simulink model "Mooventure2016_Rev5"  (Simulink 7.7)
settings: Solver=FixedStepDiscrete  StartTime=0.0  StopTime=10  RelTol=1e-3
PreLoadFcn:
  | try, eval([bdroot '_setup']); catch, eval('model_setup', ''); end
InitFcn:
  | try, eval([bdroot '_setup']); catch, eval('model_setup', ''); end
undefined symbols (not defined in the file): ECM, H1, motohawk_build_version, motohawk_trunc_name, motohawk_vardec_config_group, motohawk_vardec_path, xD
libraries: MotoHawk_lib x976, motohawk_control_primitives_lib x41, simulink x27, motohawk_annotations_lib x3
(part 2 of 16)

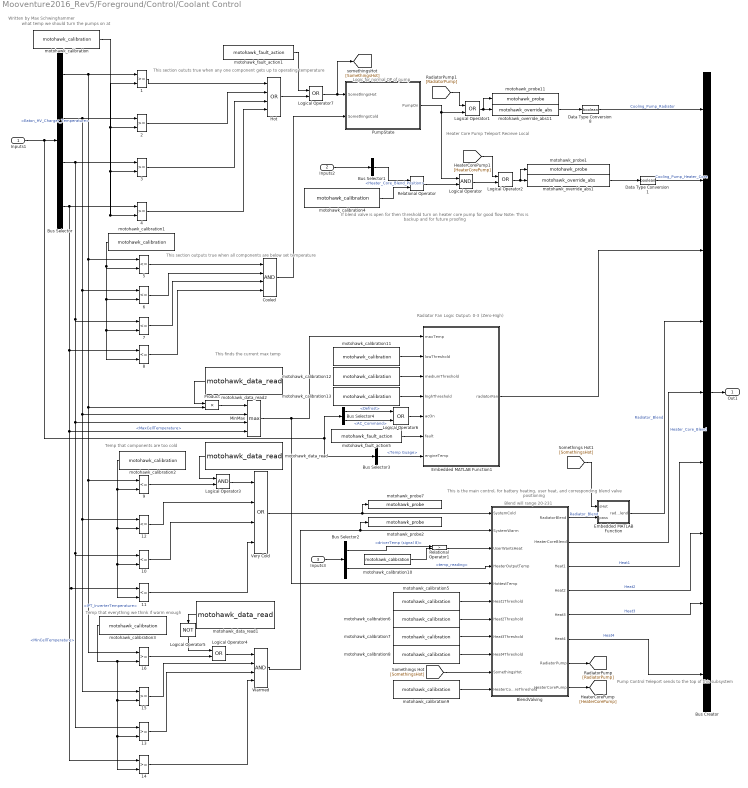
== system Mooventure2016_Rev5/Foreground/Control/Coolant Control ==
  note: This finds the current max temp
  note: Blend will range 20-231
  note: This is the main control, for battery heating, user heat,
      |  and corresponding blend valve positioning
  note: Temp that everything we think if warm enough
  note: Temp that components are too cold
  note: This section outputs true when all components
      | are below set temperature
  note: what temp we should turn the pumps on at
  note: This section oututs true when any one component
      | gets up to operating temperature
  note: Logic for normal OP of pump
  note: If blend valve is open for then threshold turn on heater
      | core pump for good flow
      | Note: This is backup and for future proofing
  note: Heater Core Pump Teleport Recieve Local
  note: Radiator Fan Logic
      | Output: 0-3 (Zero-High)
  note: Pump Control Teleport sends to the top of this subsystem
  note: Written by Max Schwinghammer
  Inputs1 : Inport
  Inputs2 : Inport  Port=2
  Inputs3 : Inport  Port=3
  {1..4,13..16} (8 alike) : RelationalOperator  OutDataTypeStr=boolean
  {5..12} (8 alike) : RelationalOperator  Operator=<=  OutDataTypeStr=boolean
  BlendValving : Stateflow chart  TreatAsAtomicUnit=on
  Bus Creator : BusCreator  Inputs=9
  Bus Selector : BusSelector  OutputSignals=Eaton_Charger.Eaton_Charger.Eaton_HV_Charger_Temperature,IPT.ID 278 IPT Status 1.IPT_InverterTemperature,Battery_Inputs.MinCellTemperature,Battery_Inputs.MaxCellTemperature
  Bus Selector1 : BusSelector  OutputSignals=Analog_Inputs.Coolant.Heater_Core_Blend_Position
  Bus Selector2 : BusSelector  OutputSignals=Driver Inputs.driverTemp (signal 8),Analog_Inputs.Coolant.temp_reading
  Bus Selector3 : BusSelector  OutputSignals=Engine Inputs.Temp Guage
  Bus Selector4 : BusSelector  OutputSignals=CAN Gateway.Defrost,CAN Gateway.AC_Command
  Cooled : Logic  Inputs=4  AllPortsSameDT=off  OutDataTypeStr=boolean
  Data Type Conversion1 : DataTypeConversion  OutDataTypeStr=boolean
  Data Type Conversion8 : DataTypeConversion  OutDataTypeStr=boolean
  Embedded MATLAB Function : Stateflow chart  TreatAsAtomicUnit=on
  Embedded MATLAB Function1 : Stateflow chart  TreatAsAtomicUnit=on
  Hot : Logic  Operator=OR  Inputs=4  AllPortsSameDT=off  OutDataTypeStr=boolean
  Logical Operator : Logic  AllPortsSameDT=off  OutDataTypeStr=boolean
  Logical Operator{1..2,4,6..7} (5 alike) : Logic  Operator=OR  AllPortsSameDT=off  OutDataTypeStr=boolean
  Logical Operator3 : Logic  AllPortsSameDT=off  OutDataTypeStr=boolean
  Logical Operator5 : Logic  Operator=NOT  Inputs=1  AllPortsSameDT=off  OutDataTypeStr=boolean
  MinMax : MinMax  Function=max  Inputs=4
  Product : Product  RndMeth=Zero
  PumpState : Stateflow chart  TreatAsAtomicUnit=on
  Relational Operator : RelationalOperator  OutDataTypeStr=boolean
  Relational Operator1 : RelationalOperator  Operator=>  OutDataTypeStr=boolean
  Very Cold : Logic  Operator=OR  Inputs=4  AllPortsSameDT=off  OutDataTypeStr=boolean
  Warmed : Logic  Inputs=4  AllPortsSameDT=off  OutDataTypeStr=boolean
  motohawk_calibration : MotoHawk_lib/Calibration & Probing Blocks/motohawk_calibration  nam='Pump_On_Temp'  val=30  storage=Calibration  show_more=off  name_source=Use Parameter  data_type=Inherit from 'Default Value'  read_level=1  write_level=1  ovr_cals=on  view_as=Number  enum_struct={'Disabled', 'Enabled'}  vector_style=Wide Row  use_help_units=off  help=''  units=''  use_header_enum=off  row_header_enum={}  col_header_enum={}  use_min_max=off  min_val=-inf  max_val=inf  use_precision=off  precision=''  gain=1  offset=0  exp=1  use_mototune_group=off  mototune_group=motohawk_vardec_path(gcb)
  motohawk_calibration1 : MotoHawk_lib/Calibration & Probing Blocks/motohawk_calibration  nam='Pump_Off_Temp'  val=25  storage=Calibration  show_more=off  name_source=Use Parameter  data_type=Inherit from 'Default Value'  read_level=1  write_level=1  ovr_cals=on  view_as=Number  enum_struct={'Disabled', 'Enabled'}  vector_style=Wide Row  use_help_units=off  help=''  units=''  use_header_enum=off  row_header_enum={}  col_header_enum={}  use_min_max=off  min_val=-inf  max_val=inf  use_precision=off  precision=''  gain=1  offset=0  exp=1  use_mototune_group=off  mototune_group=motohawk_vardec_path(gcb)
  motohawk_calibration10 : MotoHawk_lib/Calibration & Probing Blocks/motohawk_calibration  nam='Heat_On_Driver_Threshold'  val=72  storage=Calibration  show_more=off  name_source=Use Parameter  data_type=Inherit from 'Default Value'  read_level=1  write_level=1  ovr_cals=on  view_as=Number  enum_struct={'Disabled', 'Enabled'}  vector_style=Wide Row  use_help_units=off  help=''  units=''  use_header_enum=off  row_header_enum={}  col_header_enum={}  use_min_max=off  min_val=-inf  max_val=inf  use_precision=off  precision=''  gain=1  offset=0  exp=1  use_mototune_group=off  mototune_group=motohawk_vardec_path(gcb)
  motohawk_calibration11 : MotoHawk_lib/Calibration & Probing Blocks/motohawk_calibration  nam='Low_Threshold'  val=40  storage=Calibration  show_more=on  name_source=Use Parameter  data_type=double  read_level=1  write_level=1  ovr_cals=on  view_as=Number  enum_struct={'Disabled', 'Enabled'}  vector_style=Wide Row  use_help_units=off  help=''  units=''  use_header_enum=off  row_header_enum={}  col_header_enum={}  use_min_max=off  min_val=-inf  max_val=inf  use_precision=off  precision=''  gain=1  offset=0  exp=1  use_mototune_group=off  mototune_group=motohawk_vardec_path(gcb)
  motohawk_calibration12 : MotoHawk_lib/Calibration & Probing Blocks/motohawk_calibration  nam='Medium_Threshold'  val=50  storage=Calibration  show_more=on  name_source=Use Parameter  data_type=double  read_level=1  write_level=1  ovr_cals=on  view_as=Number  enum_struct={'Disabled', 'Enabled'}  vector_style=Wide Row  use_help_units=off  help=''  units=''  use_header_enum=off  row_header_enum={}  col_header_enum={}  use_min_max=off  min_val=-inf  max_val=inf  use_precision=off  precision=''  gain=1  offset=0  exp=1  use_mototune_group=off  mototune_group=motohawk_vardec_path(gcb)
  motohawk_calibration13 : MotoHawk_lib/Calibration & Probing Blocks/motohawk_calibration  nam='High_Threshold'  val=65  storage=Calibration  show_more=on  name_source=Use Parameter  data_type=double  read_level=1  write_level=1  ovr_cals=on  view_as=Number  enum_struct={'Disabled', 'Enabled'}  vector_style=Wide Row  use_help_units=off  help=''  units=''  use_header_enum=off  row_header_enum={}  col_header_enum={}  use_min_max=off  min_val=-inf  max_val=inf  use_precision=off  precision=''  gain=1  offset=0  exp=1  use_mototune_group=off  mototune_group=motohawk_vardec_path(gcb)
  motohawk_calibration2 : MotoHawk_lib/Calibration & Probing Blocks/motohawk_calibration  nam='Too_Cold_Temp'  val=0  storage=Calibration  show_more=off  name_source=Use Parameter  data_type=Inherit from 'Default Value'  read_level=1  write_level=1  ovr_cals=on  view_as=Number  enum_struct={'Disabled', 'Enabled'}  vector_style=Wide Row  use_help_units=off  help=''  units=''  use_header_enum=off  row_header_enum={}  col_header_enum={}  use_min_max=off  min_val=-inf  max_val=inf  use_precision=off  precision=''  gain=1  offset=0  exp=1  use_mototune_group=off  mototune_group=motohawk_vardec_path(gcb)
  motohawk_calibration3 : MotoHawk_lib/Calibration & Probing Blocks/motohawk_calibration  nam='Warmed_Up_Temp'  val=15  storage=Calibration  show_more=off  name_source=Use Parameter  data_type=Inherit from 'Default Value'  read_level=1  write_level=1  ovr_cals=on  view_as=Number  enum_struct={'Disabled', 'Enabled'}  vector_style=Wide Row  use_help_units=off  help=''  units=''  use_header_enum=off  row_header_enum={}  col_header_enum={}  use_min_max=off  min_val=-inf  max_val=inf  use_precision=off  precision=''  gain=1  offset=0  exp=1  use_mototune_group=off  mototune_group=motohawk_vardec_path(gcb)
  motohawk_calibration4 : MotoHawk_lib/Calibration & Probing Blocks/motohawk_calibration  nam='Blend_Pump_On_Threshold'  val=25  storage=Calibration  show_more=off  name_source=Use Parameter  data_type=Inherit from 'Default Value'  read_level=1  write_level=1  ovr_cals=on  view_as=Number  enum_struct={'Disabled', 'Enabled'}  vector_style=Wide Row  use_help_units=off  help=''  units=''  use_header_enum=off  row_header_enum={}  col_header_enum={}  use_min_max=off  min_val=-inf  max_val=inf  use_precision=off  precision=''  gain=1  offset=0  exp=1  use_mototune_group=off  mototune_group=motohawk_vardec_path(gcb)
  motohawk_calibration5 : MotoHawk_lib/Calibration & Probing Blocks/motohawk_calibration  nam='Heat1_Threshold'  val=-1  storage=Calibration  show_more=off  name_source=Use Parameter  data_type=Inherit from 'Default Value'  read_level=1  write_level=1  ovr_cals=on  view_as=Number  enum_struct={'Disabled', 'Enabled'}  vector_style=Wide Row  use_help_units=off  help=''  units=''  use_header_enum=off  row_header_enum={}  col_header_enum={}  use_min_max=off  min_val=-inf  max_val=inf  use_precision=off  precision=''  gain=1  offset=0  exp=1  use_mototune_group=off  mototune_group=motohawk_vardec_path(gcb)
  motohawk_calibration6 : MotoHawk_lib/Calibration & Probing Blocks/motohawk_calibration  nam='Heat2_Threshold'  val=-5  storage=Calibration  show_more=off  name_source=Use Parameter  data_type=Inherit from 'Default Value'  read_level=1  write_level=1  ovr_cals=on  view_as=Number  enum_struct={'Disabled', 'Enabled'}  vector_style=Wide Row  use_help_units=off  help=''  units=''  use_header_enum=off  row_header_enum={}  col_header_enum={}  use_min_max=off  min_val=-inf  max_val=inf  use_precision=off  precision=''  gain=1  offset=0  exp=1  use_mototune_group=off  mototune_group=motohawk_vardec_path(gcb)
  motohawk_calibration7 : MotoHawk_lib/Calibration & Probing Blocks/motohawk_calibration  nam='Heat3_Threshold'  val=-10  storage=Calibration  show_more=off  name_source=Use Parameter  data_type=Inherit from 'Default Value'  read_level=1  write_level=1  ovr_cals=on  view_as=Number  enum_struct={'Disabled', 'Enabled'}  vector_style=Wide Row  use_help_units=off  help=''  units=''  use_header_enum=off  row_header_enum={}  col_header_enum={}  use_min_max=off  min_val=-inf  max_val=inf  use_precision=off  precision=''  gain=1  offset=0  exp=1  use_mototune_group=off  mototune_group=motohawk_vardec_path(gcb)
  motohawk_calibration8 : MotoHawk_lib/Calibration & Probing Blocks/motohawk_calibration  nam='Heat4_Threshold'  val=-15  storage=Calibration  show_more=off  name_source=Use Parameter  data_type=Inherit from 'Default Value'  read_level=1  write_level=1  ovr_cals=on  view_as=Number  enum_struct={'Disabled', 'Enabled'}  vector_style=Wide Row  use_help_units=off  help=''  units=''  use_header_enum=off  row_header_enum={}  col_header_enum={}  use_min_max=off  min_val=-inf  max_val=inf  use_precision=off  precision=''  gain=1  offset=0  exp=1  use_mototune_group=off  mototune_group=motohawk_vardec_path(gcb)
  motohawk_calibration9 : MotoHawk_lib/Calibration & Probing Blocks/motohawk_calibration  nam='Heater_Core_Threshold'  val=46  storage=Calibration  show_more=off  name_source=Use Parameter  data_type=Inherit from 'Default Value'  read_level=1  write_level=1  ovr_cals=on  view_as=Number  enum_struct={'Disabled', 'Enabled'}  vector_style=Wide Row  use_help_units=off  help=''  units=''  use_header_enum=off  row_header_enum={}  col_header_enum={}  use_min_max=off  min_val=-inf  max_val=inf  use_precision=off  precision=''  gain=1  offset=0  exp=1  use_mototune_group=off  mototune_group=motohawk_vardec_path(gcb)
  motohawk_data_read : MotoHawk_lib/Data Storage Blocks/motohawk_data_read  source=Lookup By Name  structure=Scalar  operation=Read scalar from location by index  sz_vec=4  sz_row=2  sz_col=3  typ=boolean  nam='Eaton_Plugged_In'  checkNull=on  struct_inst_name='MyData'  struct_nam='MyStruct'
  motohawk_data_read1 : MotoHawk_lib/Data Storage Blocks/motohawk_data_read  source=Lookup By Name  structure=Scalar  operation=Read scalar from location by index  sz_vec=4  sz_row=2  sz_col=3  typ=boolean  nam='Eaton_Plugged_In'  checkNull=on  struct_inst_name='MyData'  struct_nam='MyStruct'
  motohawk_data_read2 : MotoHawk_lib/Data Storage Blocks/motohawk_data_read  source=Lookup By Name  structure=Scalar  operation=Read scalar from location by index  sz_vec=4  sz_row=2  sz_col=3  typ=boolean  nam='Eaton_Plugged_In'  checkNull=on  struct_inst_name='MyData'  struct_nam='MyStruct'
  motohawk_fault_action1 : MotoHawk_lib/Fault Management Blocks/motohawk_fault_action  nam='Pump_On'  output_status=on  eval_nam=Pump_On
  motohawk_fault_action5 : MotoHawk_lib/Fault Management Blocks/motohawk_fault_action  nam='Cooling_Max'  output_status=on  eval_nam=Cooling_Max
  motohawk_override_abs1 : MotoHawk_lib/Calibration & Probing Blocks/motohawk_override_abs  SystemSampleTime=-1  parent_name='Cooling_Pump_Heater_Core_Ovr'  parent_val=0  show_more=on  name_source=Use Parameter  parent_read_level=1  parent_override_level=1  view_as=Number  enum_struct={'Disabled', 'Enabled'}  use_help_units=off  parent_help=''  parent_units=''  use_min_max=off  parent_min=-inf  parent_max=inf  use_precision=off  parent_precision=''  parent_gain=1  parent_offset=0  parent_exp=1  use_mototune_group=off  parent_group=motohawk_vardec_path(gcb)
  motohawk_override_abs11 : MotoHawk_lib/Calibration & Probing Blocks/motohawk_override_abs  SystemSampleTime=-1  parent_name='Cooling_Pump_Radiator_Ovr'  parent_val=0  show_more=on  name_source=Use Parameter  parent_read_level=1  parent_override_level=1  view_as=Number  enum_struct={'Disabled', 'Enabled'}  use_help_units=off  parent_help=''  parent_units=''  use_min_max=off  parent_min=-inf  parent_max=inf  use_precision=off  parent_precision=''  parent_gain=1  parent_offset=0  parent_exp=1  use_mototune_group=off  parent_group=motohawk_vardec_path(gcb)
  motohawk_probe1 : MotoHawk_lib/Calibration & Probing Blocks/motohawk_probe  nam='Cooling_Pump_Heater_Core_Probe'  show_more=on  name_source=Use Parameter  read_level=1  view_as=Number  enum_struct={'Disabled', 'Enabled'}  vector_style=Wide Row  use_help_units=off  help=''  units=''  use_header_enum=off  row_header_enum={}  col_header_enum={}  use_precision=off  precision=''  gain=1  offset=0  exp=1  use_mototune_group=off  mototune_group=motohawk_vardec_path(gcb)
  motohawk_probe11 : MotoHawk_lib/Calibration & Probing Blocks/motohawk_probe  nam='Cooling_Pump_Radiator_Probe'  show_more=on  name_source=Use Parameter  read_level=1  view_as=Number  enum_struct={'Disabled', 'Enabled'}  vector_style=Wide Row  use_help_units=off  help=''  units=''  use_header_enum=off  row_header_enum={}  col_header_enum={}  use_precision=off  precision=''  gain=1  offset=0  exp=1  use_mototune_group=off  mototune_group=motohawk_vardec_path(gcb)
  motohawk_probe2 : MotoHawk_lib/Calibration & Probing Blocks/motohawk_probe  nam='System_Warm_Prb'  show_more=off  name_source=Use Parameter  read_level=1  view_as=Number  enum_struct={'Disabled', 'Enabled'}  vector_style=Wide Row  use_help_units=off  help=''  units=''  use_header_enum=off  row_header_enum={}  col_header_enum={}  use_precision=off  precision=''  gain=1  offset=0  exp=1  use_mototune_group=off  mototune_group=motohawk_vardec_path(gcb)
  motohawk_probe7 : MotoHawk_lib/Calibration & Probing Blocks/motohawk_probe  nam='System_Cold_Prb'  show_more=off  name_source=Use Parameter  read_level=1  view_as=Number  enum_struct={'Disabled', 'Enabled'}  vector_style=Wide Row  use_help_units=off  help=''  units=''  use_header_enum=off  row_header_enum={}  col_header_enum={}  use_precision=off  precision=''  gain=1  offset=0  exp=1  use_mototune_group=off  mototune_group=motohawk_vardec_path(gcb)
  Out1 : Outport
  wires:
  Inputs1/1 -> Bus Selector/1, Bus Selector3/1, Bus Selector4/1
  Bus Selector/1 -> 1/1, 5/1, 16/1, 9/1, Product/2  "<Eaton_HV_Charger_Temperature>"
  Bus Selector/2 -> 2/1, 6/1, 12/1, 15/1, MinMax/2  "<IPT_InverterTemperature>"
  Bus Selector/3 -> 3/1, 7/1, 10/1, 13/1, MinMax/3  "<MinCellTemperature>"
  Bus Selector/4 -> 4/1, 8/1, 11/1, 14/1, MinMax/4  "<MaxCellTemperature>"
  motohawk_calibration/1 -> 4/2, 3/2, 2/2, 1/2
  1/1 -> Hot/1
  2/1 -> Hot/2
  3/1 -> Hot/3
  4/1 -> Hot/4
  5/1 -> Cooled/1
  6/1 -> Cooled/2
  7/1 -> Cooled/3
  8/1 -> Cooled/4
  motohawk_calibration1/1 -> 5/2, 6/2, 7/2, 8/2
  motohawk_override_abs11/1 -> Data Type Conversion8/1
  PumpState/1(PumpOn) -> Logical Operator/1, Logical Operator1/2
  Data Type Conversion8/1 -> Bus Creator/1  "Cooling_Pump_Radiator"
  Cooled/1 -> PumpState/2(SomethingsCold)
  MinMax/1 -> BlendValving/5(HottestTemp), Embedded MATLAB Function1/1(maxTemp)
  motohawk_calibration2/1 -> 9/2, 12/2, 10/2, 11/2
  12/1 -> Very Cold/2
  10/1 -> Very Cold/3
  11/1 -> Very Cold/4
  motohawk_calibration3/1 -> 16/2, 15/2, 13/2, 14/2
  15/1 -> Warmed/2
  13/1 -> Warmed/3
  14/1 -> Warmed/4
  Very Cold/1 -> BlendValving/1(SystemCold), motohawk_probe7/1
  Warmed/1 -> BlendValving/2(SystemWarm), motohawk_probe2/1
  motohawk_override_abs1/1 -> Data Type Conversion1/1
  Data Type Conversion1/1 -> Bus Creator/2  "Cooling_Pump_Heater_Core"
  Inputs2/1 -> Bus Selector1/1
  Relational Operator/1 -> Logical Operator/2
  motohawk_calibration4/1 -> Relational Operator/2
  Bus Selector1/1 -> Relational Operator/1  "<Heater_Core_Blend_Position>"
  [SomethingsHot] -> BlendValving/10(SomethingsHot)
  motohawk_calibration5/1 -> BlendValving/6(Heat1Threshold)
  motohawk_calibration6/1 -> BlendValving/7(Heat2Threshold)
  motohawk_calibration7/1 -> BlendValving/8(Heat3Threshold)
  motohawk_calibration8/1 -> BlendValving/9(Heat4Threshold)
  Bus Selector2/2 -> BlendValving/4(HeaterOutputTemp)  "<temp_reading>"
  Inputs3/1 -> Bus Selector2/1
  motohawk_calibration9/1 -> BlendValving/11(HeaterCoreThreshold)
  Logical Operator1/1 -> motohawk_override_abs11/1, motohawk_probe11/1
  Logical Operator2/1 -> motohawk_override_abs1/1, motohawk_probe1/1
  Logical Operator/1 -> Logical Operator2/2
  BlendValving/8(HeaterCorePump) -> [HeaterCorePump]
  BlendValving/7(RadiatorPump) -> [RadiatorPump]
  [RadiatorPump] -> Logical Operator1/1
  [HeaterCorePump] -> Logical Operator2/1
  BlendValving/2(HeaterCoreBlend) -> Bus Creator/5  "Heater_Core_Blend"
  Bus Creator/1 -> Out1/1
  BlendValving/6(Heat4) -> Bus Creator/9  "Heat4"
  BlendValving/5(Heat3) -> Bus Creator/8  "Heat3"
  BlendValving/4(Heat2) -> Bus Creator/7  "Heat2"
  BlendValving/3(Heat1) -> Bus Creator/6  "Heat1"
  Logical Operator3/1 -> Very Cold/1
  9/1 -> Logical Operator3/2
  motohawk_data_read/1 -> Logical Operator3/1
  Logical Operator4/1 -> Warmed/1
  16/1 -> Logical Operator4/2
  motohawk_data_read1/1 -> Logical Operator5/1
  Logical Operator5/1 -> Logical Operator4/1
  motohawk_calibration11/1 -> Embedded MATLAB Function1/2(lowThreshold)
  motohawk_calibration12/1 -> Embedded MATLAB Function1/3(mediumThreshold)
  motohawk_calibration13/1 -> Embedded MATLAB Function1/4(highThreshold)
  Logical Operator6/1 -> Embedded MATLAB Function1/5(acOn)
  Embedded MATLAB Function1/1(radiatorFan) -> Bus Creator/3
  Relational Operator1/1 -> BlendValving/3(UserWantsHeat)
  Bus Selector2/1 -> Relational Operator1/1  "<driverTemp (signal 8)>"
  motohawk_calibration10/1 -> Relational Operator1/2
  motohawk_fault_action5/1 -> Embedded MATLAB Function1/6(fault)
  Hot/1 -> Logical Operator7/2
  Logical Operator7/1 -> PumpState/1(SomethingsHot), [SomethingsHot]
  motohawk_fault_action1/1 -> Logical Operator7/1
  BlendValving/1(RadiatorBlend) -> Embedded MATLAB Function/2(pass)  "Radiator_Blend"
  Embedded MATLAB Function/1(radBlend) -> Bus Creator/4  "Radiator_Blend"
  [SomethingsHot] -> Embedded MATLAB Function/1(sHot)
  Product/1 -> MinMax/1
  motohawk_data_read2/1 -> Product/1
  Bus Selector3/1 -> Embedded MATLAB Function1/7(engineTemp)  "<Temp Guage>"
  Bus Selector4/1 -> Logical Operator6/1  "<Defrost>"
  Bus Selector4/2 -> Logical Operator6/2  "<AC_Command>"

== system Mooventure2016_Rev5/Foreground/Control/Engine Control ==
  In1 : Inport
  Bus Creator : BusCreator
  Bus Selector : BusSelector  OutputSignals=Battery_Inputs.StateOfCharge,IPT.ID 260 IPT Status 2.IPT_MotorSpeed,Engine Inputs.Temp Guage
  Bus Selector1 : BusSelector  OutputSignals=Engine Inputs.Engine On,Engine Inputs.RPM
  Chart : Stateflow chart  TreatAsAtomicUnit=on
  Data Type Conversion{,1..5} (6 alike) : DataTypeConversion
  Engine States : Subsystem
  Product : Product  RndMeth=Zero
  SOC States : Subsystem
  Vehicle Speed States : Subsystem
  motohawk_calibration : MotoHawk_lib/Calibration & Probing Blocks/motohawk_calibration  nam='Coolant_Cold'  val=20  storage=Calibration  show_more=off  name_source=Use Parameter  data_type=Inherit from 'Default Value'  read_level=1  write_level=1  ovr_cals=on  view_as=Number  enum_struct={'Disabled', 'Enabled'}  vector_style=Wide Row  use_help_units=off  help=''  units=''  use_header_enum=off  row_header_enum={}  col_header_enum={}  use_min_max=off  min_val=-inf  max_val=inf  use_precision=off  precision=''  gain=1  offset=0  exp=1  use_mototune_group=off  mototune_group=motohawk_vardec_path(gcb)
  motohawk_calibration1 : MotoHawk_lib/Calibration & Probing Blocks/motohawk_calibration  nam='Coolant_Warm'  val=40  storage=Calibration  show_more=off  name_source=Use Parameter  data_type=Inherit from 'Default Value'  read_level=1  write_level=1  ovr_cals=on  view_as=Number  enum_struct={'Disabled', 'Enabled'}  vector_style=Wide Row  use_help_units=off  help=''  units=''  use_header_enum=off  row_header_enum={}  col_header_enum={}  use_min_max=off  min_val=-inf  max_val=inf  use_precision=off  precision=''  gain=1  offset=0  exp=1  use_mototune_group=off  mototune_group=motohawk_vardec_path(gcb)
  motohawk_calibration2 : MotoHawk_lib/Calibration & Probing Blocks/motohawk_calibration  nam='Coolant_Hot'  val=60  storage=Calibration  show_more=off  name_source=Use Parameter  data_type=Inherit from 'Default Value'  read_level=1  write_level=1  ovr_cals=on  view_as=Number  enum_struct={'Disabled', 'Enabled'}  vector_style=Wide Row  use_help_units=off  help=''  units=''  use_header_enum=off  row_header_enum={}  col_header_enum={}  use_min_max=off  min_val=-inf  max_val=inf  use_precision=off  precision=''  gain=1  offset=0  exp=1  use_mototune_group=off  mototune_group=motohawk_vardec_path(gcb)
  motohawk_calibration3 : MotoHawk_lib/Calibration & Probing Blocks/motohawk_calibration  nam='Low_RPM'  val=2400  storage=Calibration  show_more=off  name_source=Use Parameter  data_type=Inherit from 'Default Value'  read_level=1  write_level=1  ovr_cals=on  view_as=Number  enum_struct={'Disabled', 'Enabled'}  vector_style=Wide Row  use_help_units=off  help=''  units=''  use_header_enum=off  row_header_enum={}  col_header_enum={}  use_min_max=off  min_val=-inf  max_val=inf  use_precision=off  precision=''  gain=1  offset=0  exp=1  use_mototune_group=off  mototune_group=motohawk_vardec_path(gcb)
  motohawk_calibration4 : MotoHawk_lib/Calibration & Probing Blocks/motohawk_calibration  nam='Medium_RPM'  val=2800  storage=Calibration  show_more=off  name_source=Use Parameter  data_type=Inherit from 'Default Value'  read_level=1  write_level=1  ovr_cals=on  view_as=Number  enum_struct={'Disabled', 'Enabled'}  vector_style=Wide Row  use_help_units=off  help=''  units=''  use_header_enum=off  row_header_enum={}  col_header_enum={}  use_min_max=off  min_val=-inf  max_val=inf  use_precision=off  precision=''  gain=1  offset=0  exp=1  use_mototune_group=off  mototune_group=motohawk_vardec_path(gcb)
  motohawk_calibration5 : MotoHawk_lib/Calibration & Probing Blocks/motohawk_calibration  nam='High_RPM'  val=3800  storage=Calibration  show_more=off  name_source=Use Parameter  data_type=Inherit from 'Default Value'  read_level=1  write_level=1  ovr_cals=on  view_as=Number  enum_struct={'Disabled', 'Enabled'}  vector_style=Wide Row  use_help_units=off  help=''  units=''  use_header_enum=off  row_header_enum={}  col_header_enum={}  use_min_max=off  min_val=-inf  max_val=inf  use_precision=off  precision=''  gain=1  offset=0  exp=1  use_mototune_group=off  mototune_group=motohawk_vardec_path(gcb)
  motohawk_calibration6 : MotoHawk_lib/Calibration & Probing Blocks/motohawk_calibration  nam='Low_Throttle'  val=45  storage=Calibration  show_more=off  name_source=Use Parameter  data_type=Inherit from 'Default Value'  read_level=1  write_level=1  ovr_cals=on  view_as=Number  enum_struct={'Disabled', 'Enabled'}  vector_style=Wide Row  use_help_units=off  help=''  units=''  use_header_enum=off  row_header_enum={}  col_header_enum={}  use_min_max=off  min_val=-inf  max_val=inf  use_precision=off  precision=''  gain=1  offset=0  exp=1  use_mototune_group=off  mototune_group=motohawk_vardec_path(gcb)
  motohawk_calibration7 : MotoHawk_lib/Calibration & Probing Blocks/motohawk_calibration  nam='RPM_to_Wheel_Speed_Multiplier4'  val=0.01001896  storage=Calibration  show_more=off  name_source=Use Parameter  data_type=Inherit from 'Default Value'  read_level=1  write_level=1  ovr_cals=on  view_as=Number  enum_struct={'Disabled', 'Enabled'}  vector_style=Wide Row  use_help_units=off  help=''  units=''  use_header_enum=off  row_header_enum={}  col_header_enum={}  use_min_max=off  min_val=-inf  max_val=inf  use_precision=off  precision=''  gain=1  offset=0  exp=1  use_mototune_group=off  mototune_group=motohawk_vardec_path(gcb)
  motohawk_calibration8 : MotoHawk_lib/Calibration & Probing Blocks/motohawk_calibration  nam='Medium_Throttle'  val=65  storage=Calibration  show_more=off  name_source=Use Parameter  data_type=Inherit from 'Default Value'  read_level=1  write_level=1  ovr_cals=on  view_as=Number  enum_struct={'Disabled', 'Enabled'}  vector_style=Wide Row  use_help_units=off  help=''  units=''  use_header_enum=off  row_header_enum={}  col_header_enum={}  use_min_max=off  min_val=-inf  max_val=inf  use_precision=off  precision=''  gain=1  offset=0  exp=1  use_mototune_group=off  mototune_group=motohawk_vardec_path(gcb)
  motohawk_calibration9 : MotoHawk_lib/Calibration & Probing Blocks/motohawk_calibration  nam='High_Throttle'  val=100  storage=Calibration  show_more=off  name_source=Use Parameter  data_type=Inherit from 'Default Value'  read_level=1  write_level=1  ovr_cals=on  view_as=Number  enum_struct={'Disabled', 'Enabled'}  vector_style=Wide Row  use_help_units=off  help=''  units=''  use_header_enum=off  row_header_enum={}  col_header_enum={}  use_min_max=off  min_val=-inf  max_val=inf  use_precision=off  precision=''  gain=1  offset=0  exp=1  use_mototune_group=off  mototune_group=motohawk_vardec_path(gcb)
  motohawk_override_abs1 : MotoHawk_lib/Calibration & Probing Blocks/motohawk_override_abs  SystemSampleTime=-1  parent_name='Genset_Load_Ovr'  parent_val=0  show_more=off  name_source=Use Parameter  parent_read_level=1  parent_override_level=1  view_as=Number  enum_struct={'Disabled', 'Enabled'}  use_help_units=off  parent_help=''  parent_units=''  use_min_max=off  parent_min=-inf  parent_max=inf  use_precision=off  parent_precision=''  parent_gain=1  parent_offset=0  parent_exp=1  use_mototune_group=off  parent_group=motohawk_vardec_path(gcb)
  motohawk_override_abs2 : MotoHawk_lib/Calibration & Probing Blocks/motohawk_override_abs  SystemSampleTime=-1  parent_name='Genset_Enable_Ovr'  parent_val=0  show_more=off  name_source=Use Parameter  parent_read_level=1  parent_override_level=1  view_as=Number  enum_struct={'Disabled', 'Enabled'}  use_help_units=off  parent_help=''  parent_units=''  use_min_max=off  parent_min=-inf  parent_max=inf  use_precision=off  parent_precision=''  parent_gain=1  parent_offset=0  parent_exp=1  use_mototune_group=off  parent_group=motohawk_vardec_path(gcb)
  motohawk_override_abs3 : MotoHawk_lib/Calibration & Probing Blocks/motohawk_override_abs  SystemSampleTime=-1  parent_name='Genset_RPM_Ovr'  parent_val=0  show_more=off  name_source=Use Parameter  parent_read_level=1  parent_override_level=1  view_as=Number  enum_struct={'Disabled', 'Enabled'}  use_help_units=off  parent_help=''  parent_units=''  use_min_max=off  parent_min=-inf  parent_max=inf  use_precision=off  parent_precision=''  parent_gain=1  parent_offset=0  parent_exp=1  use_mototune_group=off  parent_group=motohawk_vardec_path(gcb)
  motohawk_override_abs4 : MotoHawk_lib/Calibration & Probing Blocks/motohawk_override_abs  SystemSampleTime=-1  parent_name='Genset_Throttle_Ovr'  parent_val=0  show_more=off  name_source=Use Parameter  parent_read_level=1  parent_override_level=1  view_as=Number  enum_struct={'Disabled', 'Enabled'}  use_help_units=off  parent_help=''  parent_units=''  use_min_max=off  parent_min=-inf  parent_max=inf  use_precision=off  parent_precision=''  parent_gain=1  parent_offset=0  parent_exp=1  use_mototune_group=off  parent_group=motohawk_vardec_path(gcb)
  motohawk_probe1 : MotoHawk_lib/Calibration & Probing Blocks/motohawk_probe  nam='Genset_Load_Prb'  show_more=off  name_source=Use Parameter  read_level=1  view_as=Number  enum_struct={'Disabled', 'Enabled'}  vector_style=Wide Row  use_help_units=off  help=''  units=''  use_header_enum=off  row_header_enum={}  col_header_enum={}  use_precision=off  precision=''  gain=1  offset=0  exp=1  use_mototune_group=off  mototune_group=motohawk_vardec_path(gcb)
  motohawk_probe2 : MotoHawk_lib/Calibration & Probing Blocks/motohawk_probe  nam='Genset_Enable_Prb'  show_more=off  name_source=Use Parameter  read_level=1  view_as=Number  enum_struct={'Disabled', 'Enabled'}  vector_style=Wide Row  use_help_units=off  help=''  units=''  use_header_enum=off  row_header_enum={}  col_header_enum={}  use_precision=off  precision=''  gain=1  offset=0  exp=1  use_mototune_group=off  mototune_group=motohawk_vardec_path(gcb)
  motohawk_probe3 : MotoHawk_lib/Calibration & Probing Blocks/motohawk_probe  nam='Genset_RPM_Prb'  show_more=off  name_source=Use Parameter  read_level=1  view_as=Number  enum_struct={'Disabled', 'Enabled'}  vector_style=Wide Row  use_help_units=off  help=''  units=''  use_header_enum=off  row_header_enum={}  col_header_enum={}  use_precision=off  precision=''  gain=1  offset=0  exp=1  use_mototune_group=off  mototune_group=motohawk_vardec_path(gcb)
  motohawk_probe4 : MotoHawk_lib/Calibration & Probing Blocks/motohawk_probe  nam='Genset_Throttle_Prb'  show_more=off  name_source=Use Parameter  read_level=1  view_as=Number  enum_struct={'Disabled', 'Enabled'}  vector_style=Wide Row  use_help_units=off  help=''  units=''  use_header_enum=off  row_header_enum={}  col_header_enum={}  use_precision=off  precision=''  gain=1  offset=0  exp=1  use_mototune_group=off  mototune_group=motohawk_vardec_path(gcb)
  Out1 : Outport
  wires:
  In1/1 -> Bus Selector/1, Bus Selector1/1
  Bus Selector/1 -> SOC States/1(SOC), Chart/6(SOC)  "<StateOfCharge>"
  Product/1 -> Vehicle Speed States/1(Vehicle Speed)
  motohawk_calibration7/1 -> Product/2
  SOC States/1(SOC Low) -> Data Type Conversion/1
  SOC States/2(SOC High) -> Data Type Conversion1/1
  motohawk_calibration9/1 -> Chart/16(High_Throttle)
  motohawk_calibration8/1 -> Chart/15(Medium_Throttle)
  motohawk_calibration6/1 -> Chart/14(Low_Throttle)
  motohawk_calibration5/1 -> Chart/13(High_RPM)
  motohawk_calibration4/1 -> Chart/12(Medium_RPM)
  motohawk_calibration3/1 -> Chart/11(Low_RPM)
  motohawk_calibration2/1 -> Chart/10(Coolant_Hot)
  motohawk_calibration1/1 -> Chart/9(Coolant_Warm)
  motohawk_calibration/1 -> Chart/8(Coolant_Cold)
  SOC States/3(SOC Critical) -> Data Type Conversion2/1
  Vehicle Speed States/1(Speed On) -> Data Type Conversion3/1
  Vehicle Speed States/2(Speed Off) -> Data Type Conversion4/1
  Bus Selector/2 -> Product/1  "<IPT_MotorSpeed>"
  Bus Selector/3 -> Chart/7(Coolant_Temp)  "<Temp Guage>"
  Bus Selector1/1 -> Engine States/1(Engine On)  "<Engine On>"
  Engine States/1(Engine On Out) -> Data Type Conversion5/1
  Bus Selector1/2 -> Chart/18(Engine_RPM)  "<RPM>"
  Bus Creator/1 -> Out1/1
  Chart/1(Genset_Enable) -> motohawk_override_abs2/1, motohawk_probe2/1
  Chart/2(Genset_Load) -> motohawk_override_abs1/1, motohawk_probe1/1
  Chart/3(Genset_RPM) -> motohawk_override_abs3/1, motohawk_probe3/1
  Chart/4(Genset_Throttle) -> motohawk_override_abs4/1, motohawk_probe4/1
  motohawk_override_abs4/1 -> Bus Creator/4  "Genset_Throttle"
  motohawk_override_abs3/1 -> Bus Creator/3  "Genset_RPM"
  motohawk_override_abs1/1 -> Bus Creator/2  "Genset_Load"
  motohawk_override_abs2/1 -> Bus Creator/1  "Genset_Enable"
  Data Type Conversion/1 -> Chart/1(SOC_Low)
  Data Type Conversion1/1 -> Chart/2(SOC_High)
  Data Type Conversion2/1 -> Chart/3(SOC_Critical)
  Data Type Conversion3/1 -> Chart/4(Speed_On)
  Data Type Conversion4/1 -> Chart/5(Speed_Off)
  Data Type Conversion5/1 -> Chart/17(Engine_On)

== system Mooventure2016_Rev5/Foreground/Control/Faults ==
  In1 : Inport
  Accesories : Subsystem
  Battery : Subsystem
  Freeze Frame : Subsystem
  Power Train : Subsystem
  wires:
  In1/1 -> Power Train/1(In1), Battery/1(In1), Accesories/1(In1), Freeze Frame/1(In1)

== system Mooventure2016_Rev5/Foreground/Control/Hybrid Control Code ==
  note: States:
      | 0 = SafetyMode
      | 1 = CrawlHome
      | 2 = EcoMode
      | 3 = SUVMode
  note: Determines what state to be in
  note: Written by Sarah M. Murphy
  note: IPTTorqueRequest
  Inputs : Inport
  Bus Creator : BusCreator
  CrawlHomeMode : Subsystem  TreatAsAtomicUnit=on
  Cruise Control : Subsystem
  Data Type Conversion : DataTypeConversion  OutDataTypeStr=boolean
  Data Type Conversion1 : DataTypeConversion  OutDataTypeStr=int32
  EcoMode : Subsystem  TreatAsAtomicUnit=on
  Embedded MATLAB Function : Stateflow chart  TreatAsAtomicUnit=on
  Hybrid state limits1 : Subsystem
  IPT : Subsystem
  Merge1 : Merge  Inputs=4
  Merge2 : Merge  Inputs=4
  SUVMode : Subsystem  TreatAsAtomicUnit=on
  Safety : Subsystem  TreatAsAtomicUnit=on
  Switch Case1 : SwitchCase  CaseConditions={0,1,2,3}  ShowDefaultCase=off
  Traction Control : Subsystem
  motohawk_data_def : MotoHawk_lib/Data Storage Blocks/motohawk_data_def  nam='TorqueRequest'  container_nam=''  data=0  typ=double  struct_nam='MyStruct'  storage=Volatile  outputRef=off  use_vardec=off  window=Display  read_level=1  write_level=1  ovr_cals=on  view_as=Number  enum_struct={'Disabled', 'Enabled'}  vector_style=Wide Row  use_help_units=off  help=''  units=''  use_header_enum=off  row_header_enum=''  col_header_enum=''  use_min_max=off  min_val=-inf  max_val=inf  use_precision=off  precision=''  gain=1  offset=0  exp=1  use_mototune_group=off  mototune_group=motohawk_vardec_path(gcb)  eval_name=MyData  data_stores=motohawk_sfun_data_def_data_stores  struct_instances=motohawk_sfun_data_def_struct_instances  vardecs=motohawk_sfun_data_def_vardecs
  motohawk_data_def4 : MotoHawk_lib/Data Storage Blocks/motohawk_data_def  nam='Hybrid_State'  container_nam=''  data=0  typ=int32  struct_nam='MyStruct'  storage=Volatile  outputRef=off  use_vardec=on  window=Display  read_level=1  write_level=1  ovr_cals=on  view_as=Number  enum_struct={'Disabled', 'Enabled'}  vector_style=Wide Row  use_help_units=off  help=''  units=''  use_header_enum=off  row_header_enum=''  col_header_enum=''  use_min_max=off  min_val=-inf  max_val=inf  use_precision=off  precision=''  gain=1  offset=0  exp=1  use_mototune_group=off  mototune_group=motohawk_vardec_path(gcb)  eval_name=MyData  data_stores=motohawk_sfun_data_def_data_stores  struct_instances=motohawk_sfun_data_def_struct_instances  vardecs=motohawk_sfun_data_def_vardecs
  motohawk_data_write : MotoHawk_lib/Data Storage Blocks/motohawk_data_write  source=Lookup By Name  structure=Scalar  operation=Write entire data structure at once  sz_vec=9  sz_row=2  sz_col=9  typ=double  nam='TorqueRequest'  checkNull=on  write_read_only=off  struct_inst_name=''  struct_name='MyStruct'
  motohawk_data_write3 : MotoHawk_lib/Data Storage Blocks/motohawk_data_write  source=Lookup By Name  structure=Scalar  operation=Write entire data structure at once  sz_vec=9  sz_row=2  sz_col=9  typ=int32  nam='Hybrid_State'  checkNull=on  write_read_only=off  struct_inst_name=''  struct_name='MyStruct'
  motohawk_fault_action : MotoHawk_lib/Fault Management Blocks/motohawk_fault_action  nam='Set_Crawl_Home'  output_status=on  eval_nam=Set_Crawl_Home
  motohawk_override_abs : MotoHawk_lib/Calibration & Probing Blocks/motohawk_override_abs  SystemSampleTime=-1  parent_name='HybridStateOverride'  parent_val=0  show_more=off  name_source=Use Parameter  parent_read_level=1  parent_override_level=1  view_as=Number  enum_struct={'Disabled', 'Enabled'}  use_help_units=off  parent_help=''  parent_units=''  use_min_max=off  parent_min=-inf  parent_max=inf  use_precision=off  parent_precision=''  parent_gain=1  parent_offset=0  parent_exp=1  use_mototune_group=off  parent_group=motohawk_vardec_path(gcb)
  motohawk_probe : MotoHawk_lib/Calibration & Probing Blocks/motohawk_probe  nam='HybridStateProbe'  show_more=off  name_source=Use Parameter  read_level=1  view_as=Number  enum_struct={'Disabled', 'Enabled'}  vector_style=Wide Row  use_help_units=off  help=''  units=''  use_header_enum=off  row_header_enum={}  col_header_enum={}  use_precision=off  precision=''  gain=1  offset=0  exp=1  use_mototune_group=off  mototune_group=motohawk_vardec_path(gcb)
  Outputs : Outport
  wires:
  Inputs/1 -> Safety/1(Inputs), EcoMode/1(Inputs), SUVMode/1(Inputs), CrawlHomeMode/2(Inputs), IPT/1(In1), Cruise Control/1(Inputs), Hybrid state limits1/1(Inputs)
  motohawk_override_abs/1 -> Switch Case1/1, Data Type Conversion1/1
  Switch Case1/1 -> Safety/Action
  Safety/1(Motor Torque) -> Merge1/1
  Merge1/1 -> IPT/2(In2)  "motor_Torque"
  Bus Creator/1 -> Outputs/1
  EcoMode/1(Motor Torque) -> Merge1/3
  Switch Case1/4 -> SUVMode/Action
  Switch Case1/3 -> EcoMode/Action
  CrawlHomeMode/1(Motor Torque) -> Merge1/2
  Hybrid state limits1/2(SoCBounds) -> CrawlHomeMode/1(SoCBounds)
  Merge2/1 -> Data Type Conversion/1  "motor_Enable"
  Safety/2(Motor Enable) -> Merge2/1
  EcoMode/2(Motor Enable) -> Merge2/3
  SUVMode/1(Motor Torque) -> Merge1/4
  SUVMode/2(Motor Enable) -> Merge2/4
  IPT/3(InReverse) -> SUVMode/2(InReverse), EcoMode/2(InReverse), CrawlHomeMode/3(InReverse)
  Data Type Conversion1/1 -> motohawk_data_write3/1
  Hybrid state limits1/1(state_o) -> Embedded MATLAB Function/2(current_state)  "Hybrid_State"
  Embedded MATLAB Function/1(state) -> motohawk_override_abs/1, motohawk_probe/1
  motohawk_fault_action/1 -> Embedded MATLAB Function/1(set_crawl_home)
  Switch Case1/2 -> CrawlHomeMode/Action
  CrawlHomeMode/2(Motor Enable) -> Merge2/2
  Data Type Conversion/1 -> Bus Creator/4  "motor_Enable"
  IPT/2(IPT_Direction) -> Bus Creator/3  "IPTDirection"
  Cruise Control/1(Outputs) -> Bus Creator/1  "Cruise Control"
  IPT/1(Torque_Request) -> Cruise Control/2(Torque)  "IPTTorqueRequest"
  Cruise Control/2(TorqueOut) -> Traction Control/1(In1)  "IPTTorqueRequest"
  Traction Control/1(Out1) -> Bus Creator/2, motohawk_data_write/1  "IPTTorqueRequest"

== system Mooventure2016_Rev5/Foreground/Control/Vehicle Run/Stop Determination ==
  note: Has to go to NOT because of wiring
  Inputs : Inport
  Bus Selector : BusSelector  OutputSignals=Eaton_Charger.Eaton_Charger.ChargerState
  Chart : Stateflow chart  TreatAsAtomicUnit=on
  Logical Operator : Logic  Operator=OR  Inputs=3  AllPortsSameDT=off  OutDataTypeStr=boolean
  Logical Operator1 : Logic  Operator=OR  AllPortsSameDT=off  OutDataTypeStr=boolean
  Logical Operator5 : Logic  Operator=NOT  AllPortsSameDT=off  OutDataTypeStr=boolean
  Relational Operator : RelationalOperator  OutDataTypeStr=boolean
  motohawk_calibration1 : MotoHawk_lib/Calibration & Probing Blocks/motohawk_calibration  nam='Auto_Battery_Startup'  val=0  storage=Calibration  show_more=off  name_source=Use Parameter  data_type=Inherit from 'Default Value'  read_level=1  write_level=1  ovr_cals=on  view_as=Number  enum_struct={'Disabled', 'Enabled'}  vector_style=Wide Row  use_help_units=off  help=''  units=''  use_header_enum=off  row_header_enum={}  col_header_enum={}  use_min_max=off  min_val=-inf  max_val=inf  use_precision=off  precision=''  gain=1  offset=0  exp=1  use_mototune_group=off  mototune_group=motohawk_vardec_path(gcb)
  motohawk_calibration3 : MotoHawk_lib/Calibration & Probing Blocks/motohawk_calibration  nam='Eaton_Is_Charging'  val=2  storage=Calibration  show_more=off  name_source=Use Parameter  data_type=Inherit from 'Default Value'  read_level=1  write_level=1  ovr_cals=on  view_as=Number  enum_struct={'Disabled', 'Enabled'}  vector_style=Wide Row  use_help_units=off  help=''  units=''  use_header_enum=off  row_header_enum={}  col_header_enum={}  use_min_max=off  min_val=-inf  max_val=inf  use_precision=off  precision=''  gain=1  offset=0  exp=1  use_mototune_group=off  mototune_group=motohawk_vardec_path(gcb)
  motohawk_data_read : MotoHawk_lib/Data Storage Blocks/motohawk_data_read  source=Lookup By Name  structure=Scalar  operation=Read scalar from location by index  sz_vec=4  sz_row=2  sz_col=3  typ=boolean  nam='Batt_Load_Enable'  checkNull=on  struct_inst_name='MyData'  struct_nam='MyStruct'
  motohawk_data_read1 : MotoHawk_lib/Data Storage Blocks/motohawk_data_read  source=Lookup By Name  structure=Scalar  operation=Read scalar from location by index  sz_vec=4  sz_row=2  sz_col=3  typ=boolean  nam='Shutdown_Req'  checkNull=on  struct_inst_name='MyData'  struct_nam='MyStruct'
  motohawk_data_read2 : MotoHawk_lib/Data Storage Blocks/motohawk_data_read  source=Lookup By Name  structure=Scalar  operation=Read scalar from location by index  sz_vec=4  sz_row=2  sz_col=3  typ=boolean  nam='Batt_Contactor_Status'  checkNull=on  struct_inst_name='MyData'  struct_nam='MyStruct'
  motohawk_data_write : MotoHawk_lib/Data Storage Blocks/motohawk_data_write  source=Lookup By Name  structure=Scalar  operation=Write entire data structure at once  sz_vec=9  sz_row=2  sz_col=9  typ=boolean  nam='Vehicle_Enable'  checkNull=on  write_read_only=off  struct_inst_name=''  struct_name='MyStruct'
  motohawk_data_write1 : MotoHawk_lib/Data Storage Blocks/motohawk_data_write  source=Lookup By Name  structure=Scalar  operation=Write entire data structure at once  sz_vec=9  sz_row=2  sz_col=9  typ=boolean  nam='Torque_Enable'  checkNull=on  write_read_only=off  struct_inst_name=''  struct_name='MyStruct'
  motohawk_data_write2 : MotoHawk_lib/Data Storage Blocks/motohawk_data_write  source=Lookup By Name  structure=Scalar  operation=Write entire data structure at once  sz_vec=9  sz_row=2  sz_col=9  typ=boolean  nam='Vehicle_Ready'  checkNull=on  write_read_only=off  struct_inst_name=''  struct_name='MyStruct'
  motohawk_din : MotoHawk_lib/Digital I//O Blocks/motohawk_din  resource_name='ESTOP2'  text_resource=ESTOP  code_resource=NONE  val_resource=-1  target=ECM-5554-112-0904-xD  resource_enum_str=(None)=-1,CNK=1,SPD3=2,SPD2=3,AN24=4,AN25=5,AN26=6,AN27=7,AN28=8,AN29=9,AN30=10,AN31=11,AN32=12,AN33=13,CAM=14,SPD1=15,ESTOP=16,AN1=17,AN2=18,AN3=19,AN4=20,AN5=21,AN6=22,AN7=23,AN8=24,AN9=25,AN10=26,AN11=27,AN12=28,AN13=29,AN14=30,AN15=31,AN16=32,AN17=33,AN18=34,AN19=35,AN20=36,AN21=37,AN22=38,AN23=39  pullup=None  use_stat=off  use_vardec=off  nam='DIN'  read_level=1  write_level=1  group='System | I/O Pins | Inputs Config'
  motohawk_fault_action : MotoHawk_lib/Fault Management Blocks/motohawk_fault_action  nam='Dyno_Shutdown'  output_status=on  eval_nam=Dyno_Shutdown
  Component_Keyed : Outport
  wires:
  motohawk_data_read2/1 -> Chart/3(Batt_Contactor_Status)
  Chart/4(Keyed_Relay) -> Component_Keyed/1
  Chart/1(Vehicle_Enable) -> motohawk_data_write/1
  Chart/2(Vehicle_Ready) -> motohawk_data_write2/1
  Chart/3(Torque_Enable) -> motohawk_data_write1/1
  Logical Operator/1 -> Chart/1(Shutdown)
  motohawk_data_read1/1 -> Logical Operator/3
  motohawk_fault_action/1 -> Logical Operator/2
  motohawk_din/1 -> Logical Operator5/1
  Logical Operator5/1 -> Logical Operator/1
  Inputs/1 -> Bus Selector/1
  Relational Operator/1 -> Chart/4(Charging)
  Bus Selector/1 -> Relational Operator/1  "<ChargerState>"
  motohawk_calibration3/1 -> Relational Operator/2
  Logical Operator1/1 -> Chart/2(Batt_Load_Enable)
  motohawk_data_read/1 -> Logical Operator1/1
  motohawk_calibration1/1 -> Logical Operator1/2
